simulink model "oloop3"  (Simulink 2.09)
settings: Solver=ode45  StartTime=0.0  StopTime=120  MaxStep=2  RelTol=1e-3  AbsTol=1e-3
undefined symbols (not defined in the file or in its folder): Aac, Bac, Cac, Dac
settings Model: SaveTime=off  SaveOutput=off  ConsistencyChecking=off  RTWTemplateMakefile=grt_vc.tmf

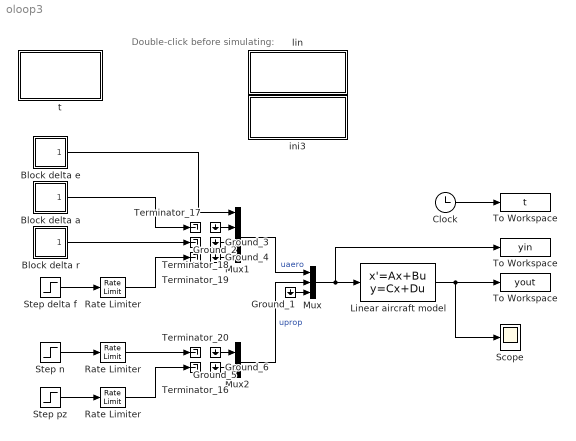
== system oloop3 ==
  note: Double-click
      | before
      | simulating:
  " Rate Limiter" : RateLimiter  RisingSlewLimit=1.0  FallingSlewLimit=-1.0
  " To Workspace  " : ToWorkspace  VariableName=yin  SampleTime=0
      settings: Buffer=1000
  Block delta a : Subsystem  mask(Block Fcn){@1=0, @2=3*pi/180, @3=0, @4=2}
      mask prompts: @1 "Initial value (=final value):"; @2 "Amplitude of block (+ = step up, - = step down):"; @3 "Start time of block:"; @4 "Stop time of block:"
      mask help: Block Function
      mask init:
      | yinit=@1; yblock=@2; tstart=@3; tstop=@4;
      mask Help: This block implements a block signal.\nDefine the initial (=final) value, the\namplitude of the block (positive\n= upwards, negative=downwards),\nthe start time, and the stop time (must\nbe smaller than the start time).
      mask Display: plot(0,0,100,100,[100,60,60,20,20,0],[50,50,89,89,50,50])
  Block delta e : Subsystem  mask(Block Fcn){@1=0, @2=3*pi/180, @3=0, @4=2}
      mask prompts: @1 "Initial value (=final value):"; @2 "Amplitude of block (+ = step up, - = step down):"; @3 "Start time of block:"; @4 "Stop time of block:"
      mask help: Block Function
      mask init:
      | yinit=@1; yblock=@2; tstart=@3; tstop=@4;
      mask Help: This block implements a block signal.\nDefine the initial (=final) value, the\namplitude of the block (positive\n= upwards, negative=downwards),\nthe start time, and the stop time (must\nbe smaller than the start time).
      mask Display: plot(0,0,100,100,[100,60,60,20,20,0],[50,50,89,89,50,50])
  Block delta r : Subsystem  mask(Block Fcn){@1=0, @2=3*pi/180, @3=0, @4=2}
      mask prompts: @1 "Initial value (=final value):"; @2 "Amplitude of block (+ = step up, - = step down):"; @3 "Start time of block:"; @4 "Stop time of block:"
      mask help: Block Function
      mask init:
      | yinit=@1; yblock=@2; tstart=@3; tstop=@4;
      mask Help: This block implements a block signal.\nDefine the initial (=final) value, the\namplitude of the block (positive\n= upwards, negative=downwards),\nthe start time, and the stop time (must\nbe smaller than the start time).
      mask Display: plot(0,0,100,100,[100,60,60,20,20,0],[50,50,89,89,50,50])
  Clock : Clock
  Ground_{1..6} (6 alike) : Ground
  Linear aircraft model : StateSpace  A=Aac  B=Bac  C=Cac  D=Dac  X0=0
  Mux : Mux  Inputs=[4 2 6]
  Mux1 : Mux  Inputs=4
  Mux2 : Mux  Inputs=2
  Rate Limiter : RateLimiter  RisingSlewLimit=3*pi/180  FallingSlewLimit=-3*pi/180
  "Rate Limiter " : RateLimiter  RisingSlewLimit=50  FallingSlewLimit=-50
  Scope : Scope
      settings: TickLabels=on  TimeRange=120.000000  YMin=-50.000000  YMax=50.000000  SaveToWorkspace=off  SaveName=ScopeData
  Step delta f : Step  Time=0.001  Before=0  After=3*pi/180
  Step n : Step  Time=1  Before=0  After=200
  Step pz : Step  Time=0.001  Before=0  After=2
  Terminator_{16..20} (5 alike) : Terminator
  To Workspace : ToWorkspace  VariableName=t  SampleTime=0
      settings: Buffer=1000
  "To Workspace " : ToWorkspace  VariableName=yout  SampleTime=0
      settings: Buffer=1000
  ini3 : Subsystem
      settings: OpenFcn=incoload
      mask Type: incoload
      mask Display: disp('1b. Load linear\nmodel from file\nINCOLOAD')
  lin : Subsystem
      settings: OpenFcn=aclin
      mask Type: linearize aircraft model
      mask Display: disp('1a. Call lineari-\nzation routine\nACLIN')
  t : Subsystem
      settings: OpenFcn=fdchelp oloop
      mask Display: disp('OLOOP3\nMarc Rauw\nOctober 1997')
  wires:
  Ground_6/1 -> Mux2/2
  Ground_5/1 -> Mux2/1
  Ground_4/1 -> Mux1/4
  Ground_3/1 -> Mux1/3
  Ground_2/1 -> Mux1/2
  Block delta e/1(block) -> Mux1/1
  Step pz/1 -> " Rate Limiter"/1
  Step n/1 -> "Rate Limiter "/1
  Step delta f/1 -> Rate Limiter/1
  Clock/1 -> To Workspace/1
  Linear aircraft model/1 -> "To Workspace "/1, Scope/1
  Mux/1 -> Linear aircraft model/1, " To Workspace  "/1
  Block delta a/1(block) -> Terminator_17/1
  Block delta r/1(block) -> Terminator_18/1
  Rate Limiter/1 -> Terminator_19/1
  "Rate Limiter "/1 -> Terminator_20/1
  " Rate Limiter"/1 -> Terminator_16/1
  Ground_1/1 -> Mux/3
  Mux2/1 -> Mux/2  "uprop"
  Mux1/1 -> Mux/1  "uaero"

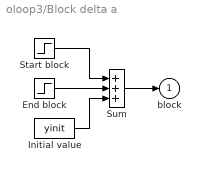
== system oloop3/Block delta a ==
  End block : Step  Time=tstop  Before=0  After=-yblock
  Initial value : Constant  Value=yinit
  Start block : Step  Time=tstart  Before=0  After=yblock
  Sum : Sum  Inputs=+++
  block : Outport  Port=1  InitialOutput=0
  wires:
  End block/1 -> Sum/2
  Start block/1 -> Sum/1
  Initial value/1 -> Sum/3
  Sum/1 -> block/1

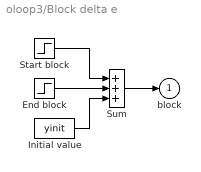
== system oloop3/Block delta e ==
  End block : Step  Time=tstop  Before=0  After=-yblock
  Initial value : Constant  Value=yinit
  Start block : Step  Time=tstart  Before=0  After=yblock
  Sum : Sum  Inputs=+++
  block : Outport  Port=1  InitialOutput=0
  wires:
  Sum/1 -> block/1
  Initial value/1 -> Sum/3
  Start block/1 -> Sum/1
  End block/1 -> Sum/2

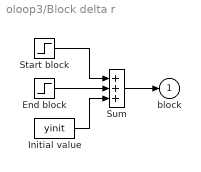
== system oloop3/Block delta r ==
  End block : Step  Time=tstop  Before=0  After=-yblock
  Initial value : Constant  Value=yinit
  Start block : Step  Time=tstart  Before=0  After=yblock
  Sum : Sum  Inputs=+++
  block : Outport  Port=1  InitialOutput=0
  wires:
  Sum/1 -> block/1
  Initial value/1 -> Sum/3
  Start block/1 -> Sum/1
  End block/1 -> Sum/2

== system oloop3/ini3 ==

== system oloop3/lin ==

== system oloop3/t ==
